simulink model "rate_delay_mdl"  (Simulink 7.0)
settings: Solver=ode4  SolverMode=SingleTasking  StartTime=0.0  StopTime=tdur  FixedStep=dt  RelTol=1e-3
values from neighbouring files (symbols this model uses):
  dt = 0.1    [rate_controller_response.m]
  I = 30000    [rate_controller_response.m]
  Kd = 1150    [rate_controller_response.m]
  Krcs = 1    [rate_controller_response.m]
  t_delay = 3    [rate_controller_response.m]
  Tdist = 0.1    [rate_controller_response.m]
  Trcs_max = 57    [rate_controller_response.m]
libraries: simulink_extras x1
settings Model: Creator=hardac_s  LastModifiedBy=hardac_s
settings DataIOCC: LimitDataPoints=off  SaveOutput=off  SignalLoggingName=sigsOut
settings DebuggingCC: SaveWithParameterizedLinksMsg=none  SignalResolutionControl=TryResolveAllWithWarning  SolverPrmCheckMsg=none  MultiTaskDSMMsg=warning  MultiTaskCondExecSysMsg=none  StrictBusMsg=None
settings HardwareCC: TargetUnknown=on
settings RTWCC: IncludeERTFirstTime=on

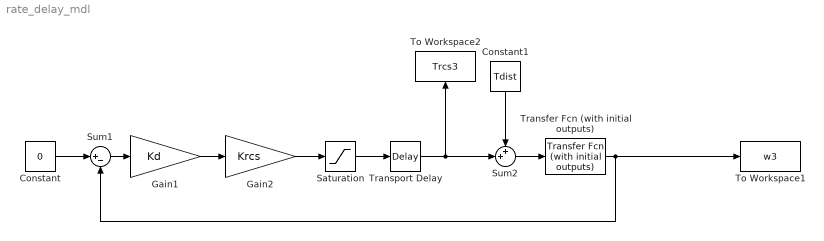
== system rate_delay_mdl ==
  Constant : Constant  Value=0  OutDataType=sfix(16)  OutScaling=2^0
  Constant1 : Constant  Orientation=down  Value=Tdist  OutDataType=sfix(16)  OutScaling=2^0
  Gain1 : Gain  Gain=Kd  ParameterDataType=sfix(16)  ParameterScaling=2^0  OutDataType=sfix(16)  OutScaling=2^0  SaturateOnIntegerOverflow=on
  Gain2 : Gain  Gain=Krcs  ParameterDataType=sfix(16)  ParameterScaling=2^0  OutDataType=sfix(16)  OutScaling=2^0  SaturateOnIntegerOverflow=on
  Saturation : Saturate  UpperLimit=Trcs_max  LowerLimit=-Trcs_max  SampleTime=dt
  Sum1 : Sum  Inputs=|+-  OutDataType=sfix(16)  OutScaling=2^0  SaturateOnIntegerOverflow=on
  Sum2 : Sum  Inputs=++|  OutDataType=sfix(16)  OutScaling=2^0  SaturateOnIntegerOverflow=on
  To Workspace1 : ToWorkspace  VariableName=w3  SampleTime=dt  SaveFormat=Array
  To Workspace2 : ToWorkspace  VariableName=Trcs3  SampleTime=dt  SaveFormat=Array
      settings: Orientation=up
  Transfer Fcn (with initial outputs) : simulink_extras/Additional Linear/Transfer Fcn (with initial outputs)  SystemSampleTime=-1  N=[1]  D=[I 0]  Y0=w0  U0=0
  Transport Delay : TransportDelay  DelayTime=t_delay
  wires:
  Constant/1 -> Sum1/1
  Sum1/1 -> Gain1/1
  Gain1/1 -> Gain2/1
  Transfer Fcn (with initial outputs)/1 -> Sum1/2, To Workspace1/1
  Sum2/1 -> Transfer Fcn (with initial outputs)/1
  Gain2/1 -> Saturation/1
  Constant1/1 -> Sum2/1
  Transport Delay/1 -> Sum2/2, To Workspace2/1
  Saturation/1 -> Transport Delay/1
